simulink model "first_order_tf"  (R2015b)
settings: Solver=ode1  StartTime=0.0  StopTime=10.0  RelTol=1e-3
values from neighbouring files (symbols this model uses):
  K = Simulink.Parameter    [first_order_tf_init.m]
  tau = Simulink.Parameter    [first_order_tf_init.m]
settings Model: Creator=C3038028  LastModifiedBy=C3038028
settings OptimizationCC: DefaultParameterBehavior=Inlined  OptimizeModelRefInitCode=on  LifeSpan=1
settings HardwareCC: TargetBitPerPointer=64  TargetLongLongMode=on  TargetIntDivRoundTo=Zero  TargetEndianess=LittleEndian  TargetWordSize=64  TargetHWDeviceType=MATLAB Host  ProdEqTarget=off
settings RTWCC: SystemTargetFile=ert_shrlib.tlc  TemplateMakefile=ert_default_tmf  Description=Embedded Coder (host-based shared library target)  BuildConfiguration=Faster Runs
settings CodeAppCC: IgnoreCustomStorageClasses=off
settings STFCustomTargetCC: GenerateSampleERTMain=on  ParMdlRefBuildCompliant=on  CompOptLevelCompliant=on  ConcurrentExecutionCompliant=off  GeneratePreprocessorConditionals=Use local settings  CombineOutputUpdateFcns=on  ERTCustomFileBanners=on  SupportNonInlinedSFcns=off  MATLABClassNameForMDSCustomization=Simulink.SoftwareTarget.ERTCustomization  ModelStepFunctionPrototypeControlCompliant=on  CPPClassGenCompliant=off  GRTInterface=off  UseToolchainInfoCompliant=on  SystemTargetFile=ert_shrlib.tlc
settings ERTTargetCC: GenerateSampleERTMain=on  ConcurrentExecutionCompliant=off  ERTFirstTimeCompliant=off  SupportContinuousTime=on  CPPClassGenCompliant=off  InlinedParameterPlacement=NonHierarchical  ERTCustomFileTemplate=example_file_process.tlc

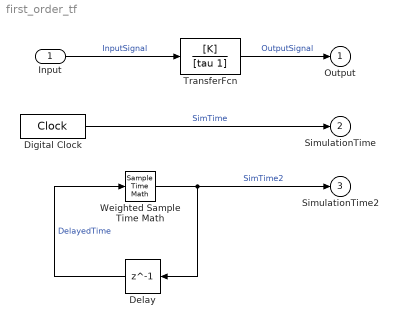
== system first_order_tf ==
  Input : Inport
  Delay : Delay  DelayLength=1
  Digital Clock : DigitalClock  SampleTime=0.01
  TransferFcn : TransferFcn  Numerator=[K]  Denominator=[tau 1]
  Weighted Sample Time Math : SampleTimeMath  weightValue=1
  Output : Outport
  SimulationTime : Outport  Port=2
  SimulationTime2 : Outport  Port=3
  wires:
  Input/1 -> TransferFcn/1  "InputSignal"
  TransferFcn/1 -> Output/1  "OutputSignal"
  Digital Clock/1 -> SimulationTime/1  "SimTime"
  Weighted Sample Time Math/1 -> SimulationTime2/1, Delay/1  "SimTime2"
  Delay/1 -> Weighted Sample Time Math/1  "DelayedTime"
